simulink model "Athena"  (R2018b)
settings: Solver=ode3  StartTime=0.0  StopTime=10  RelTol=1e-3  EnableMultiTasking=on
libraries: legoev3lib x12, Beeper x1, athenaControls x1, colorDetector x1, DistanceSensor x1, FlagLibrary x1, ManualMotor x1
settings Model: FPTRunName=Active  ExtModeTrigDuration=2  Creator=Sjoerd  LastModifiedBy=Sjoerd
settings SolverCC: PositivePriorityOrder=on
settings DataIOCC: LimitDataPoints=on  SaveFormat=Array
settings OptimizationCC: ExpressionDepthLimit=2147483647  LifeSpan=Inf  MaxStackSize=64
settings DebuggingCC: UnderspecifiedInitializationDetection=Classic  MergeDetectMultiDrivingBlocksExec=none  FcnCallInpInsideContextMsg=warning  AllowSymbolicDim=off  StateNameClashWarn=warning  SFUnexpectedBacktrackingDiag=warning  SFNoUnconditionalDefaultTransitionDiag=warning  SFExecutionAtInitializationDiag=none
settings HardwareCC: ProdBitPerPointer=32  ProdBitPerSizeT=32  ProdBitPerPtrDiffT=32  ProdLargestAtomicInteger=Long  ProdWordSize=32  ProdHWDeviceType=ARM Compatible->ARM 9  UseEmbeddedCoderFeatures=off  UseSimulinkCoderFeatures=off
settings ModelReferenceCC: PropagateSignalLabelsOutOfModel=off
settings SFSimCC: SimUseLocalCustomCode=off
settings RTWCC: SystemTargetFile=ert.tlc  HardwareBoard=LEGO MINDSTORMS EV3  TemplateMakefile=ert_default_tmf  GenerateReport=on  RTWVerbose=off  RTWUseLocalCustomCode=off  Toolchain=Sourcery G++ Lite v2009q3  BuildConfiguration=Faster Runs  LaunchReport=on
settings CodeAppCC: ForceParamTrailComments=on  OperatorAnnotations=on  StateflowObjectComments=on  MATLABSourceComments=on
settings ERTTargetCC: MultiwordLength=2048  ERTCustomFileBanners=off  SupportContinuousTime=on  SupportNonInlinedSFcns=on  RemoveResetFunc=off  SupportVariableSizeSignals=on  ModelStepFunctionPrototypeControlCompliant=off
settings ConfigComp: CovMetricSettings=dw  CovHtmlReporting=on  CovSaveCumulativeToWorkspaceVar=on  CovSaveSingleToWorkspaceVar=on  CovExternalEMLEnable=off  CovSFcnEnable=off

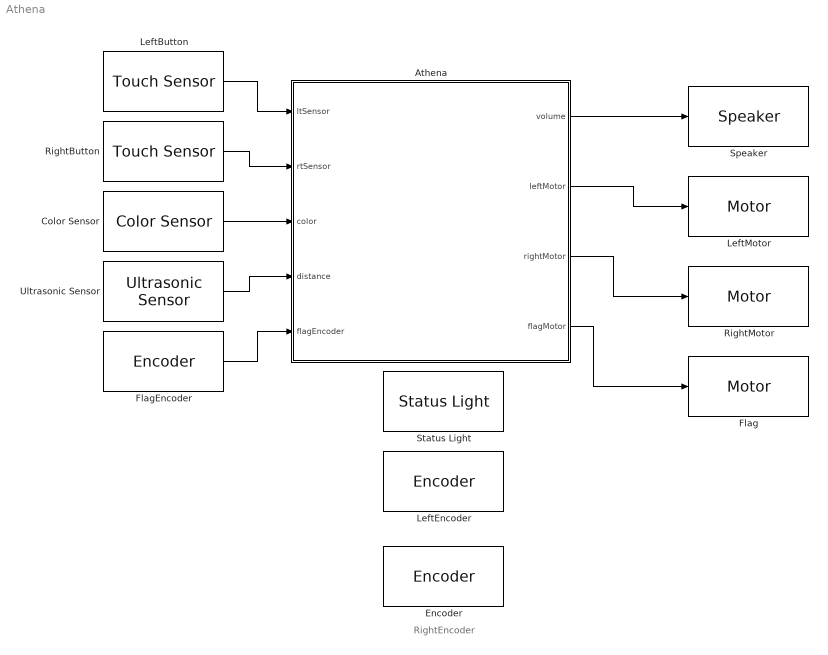
== system Athena ==
  note: RightEncoder
  Athena : Stateflow chart  TreatAsAtomicUnit=on
  Color Sensor : legoev3lib/Color Sensor  portNumber=3  mode=Color  sampleTime=0.1
      settings: SourceProductName=Simulink Support Package for LEGO MINDSTORMS EV3 Hardware  SourceProductBaseCode=LEGOEV3
  Encoder : legoev3lib/Encoder  portNumber=C  opMode=No reset  sampleTime=0.1
      settings: SourceProductName=Simulink Support Package for LEGO MINDSTORMS EV3 Hardware  SourceProductBaseCode=LEGOEV3
  Flag : legoev3lib/Motor  sportNumber=D  sstopAction=Brake
  FlagEncoder : legoev3lib/Encoder  portNumber=A  opMode=No reset  sampleTime=0.1
      settings: SourceProductName=Simulink Support Package for LEGO MINDSTORMS EV3 Hardware  SourceProductBaseCode=LEGOEV3
  LeftButton : legoev3lib/Touch Sensor  portNumber=1  sampleTime=0.1
      settings: SourceProductName=Simulink Support Package for LEGO MINDSTORMS EV3 Hardware  SourceProductBaseCode=LEGOEV3
  LeftEncoder : legoev3lib/Encoder  portNumber=B  opMode=No reset  sampleTime=0.1
      settings: SourceProductName=Simulink Support Package for LEGO MINDSTORMS EV3 Hardware  SourceProductBaseCode=LEGOEV3
  LeftMotor : legoev3lib/Motor  sportNumber=B  sstopAction=Brake
  RightButton : legoev3lib/Touch Sensor  portNumber=2  sampleTime=0.1
      settings: SourceProductName=Simulink Support Package for LEGO MINDSTORMS EV3 Hardware  SourceProductBaseCode=LEGOEV3
  RightMotor : legoev3lib/Motor  sportNumber=C  sstopAction=Brake
  Speaker : legoev3lib/Speaker  sinputMode=Volume only  sspeakerFreq=32  sspeakerVolume=50  sspeakerDuration=100
      settings: SourceProductName=Simulink Support Package for LEGO MINDSTORMS EV3 Hardware  SourceProductBaseCode=LEGOEV3
  Status Light : legoev3lib/Status Light
      settings: SourceProductName=Simulink Support Package for LEGO MINDSTORMS EV3 Hardware  SourceProductBaseCode=LEGOEV3
  Ultrasonic Sensor : legoev3lib/Ultrasonic Sensor  PortNumber=4  sampleTime=0.1
      settings: SourceProductName=Simulink Support Package for LEGO MINDSTORMS EV3 Hardware  SourceProductBaseCode=LEGOEV3
  wires:
  RightButton/1 -> Athena/2(rtSensor)
  Athena/1(volume) -> Speaker/1
  FlagEncoder/1 -> Athena/5(flagEncoder)
  Athena/3(rightMotor) -> RightMotor/1
  Athena/2(leftMotor) -> LeftMotor/1
  Color Sensor/1 -> Athena/3(color)
  Ultrasonic Sensor/1 -> Athena/4(distance)
  Athena/4(flagMotor) -> Flag/1
  LeftButton/1 -> Athena/1(ltSensor)

== stateflow chart Athena/Athena ==
  state MotorControls [parallel]
    settings: executionOrder=3
    state Autonomous
      (history)
      state Idle
        entry:
        rightMotor = 0
        leftMotor = 0
      state Turn90
      state DriveStraight
        entry:
        rightMotor = 0
        leftMotor = 0
      state FollowLine
      (default) -> Idle
      Turn90 -> Idle : [DONE_TURNING]
      Idle -> Turn90 [order 2] : [TURN]
      FollowLine -> Idle
      DriveStraight -> Idle : [DRIVE==false]
      Idle -> DriveStraight [order 1] : [DRIVE]
      Idle -> FollowLine [order 3] : [FOLLOW]
    state ManualMotor
    (default) -> ManualMotor
    ManualMotor -> MotorControls.Autonomous : [START_AUTONOMOUS]
    MotorControls.Autonomous -> ManualMotor : [STOP_AUTONOMOUS]
  state Beeper1 [parallel]
    settings: executionOrder=7
  state FlagControl [parallel]
    settings: executionOrder=6
  state TaskMaster [parallel]
    settings: executionOrder=1
    state Autonomous
      (history)
      state Step2_1
        entry:
        maxSpeed = 20
        DRIVE = true
        exit:
        DRIVE = false
      state Step2_2
        entry:
        rightMotor = 0
        leftMotor = 0
      state Step3
        state step3_1
          entry:
          BEEP = true
          TURN = true
          exit:
          BEEP = false
          TURN = false
        state Flee
          entry:
          maxSpeed = 100
          DRIVE = true
        (default) -> step3_1
        step3_1 -> Flee : [DONE_TURNING]
      state Step4
        state FoundGreen
          entry:
          BEEP = true
          RAISEFLAG = true
          exit:
          BEEP = false
          RAISEFLAG = false
        state step4_1
          entry:
          BEEP = true
          FOLLOWBLACK = true
          exit:
          BEEP = false
          FOLLOWBLACK = false
        (default) -> step4_1
        step4_1 -> FoundGreen : [GREEN]
      (default) -> Step2_1
      Step2_1 -> Step2_2 : [FOUND_BEAST]
      Step2_2 -> Step3 : after(5,sec)
      Step3 -> Step4 : [BLACK]{DRIVE=false}
    state Manual
    (default) -> Manual
    TaskMaster.Autonomous -> Manual : [STOP_AUTONOMOUS]
    Manual -> TaskMaster.Autonomous : [START_AUTONOMOUS]
  state ColorSensor [parallel]
    settings: executionOrder=5
  state DistanceSensor [parallel]
    settings: executionOrder=4
  state Buttons [parallel]
    settings: executionOrder=2
  data: FORWARD_STOP function_input; TURN_LEFT function_input; TURN_RIGHT function_input; STOP_TURNING function_input; BEEP function_input; ltSensor input; rtSensor input; volume output; leftMotor output; rightMotor output; color input; distance input; flagEncoder input; flagMotor output; STOP_AUTONOMOUS local; BEEP local; DRIVE local; FOLLOWBLACK local; RAISEFLAG local; DONE_TURNING local; BLACK local; TURN local; FORWARD_STOP local; TURN_RIGHT local; TURN_LEFT local; STOP_TURNING local; START_AUTONOMOUS local; GREEN local; FOUND_BEAST local; FOLLOW local; maxSpeed local
